simulink model "AccTarSel"  (R2018b)
settings: Solver=FixedStepDiscrete  StartTime=0.0  StopTime=inf  FixedStep=0.01  RelTol=1e-3
PostLoadFcn:
  | if any(exist('dsrtsu_mdlpostloadfcn', 'file') ~= 0), dsrtsu_mdlpostloadfcn('Execute', bdroot); end
values from neighbouring files (symbols this model uses):
  P_adtMaxBDC = 1.0    [AccTarSel.sldd]
  P_aFOCApproachIntpAcitve = -0.6    [AccTarSel.sldd]
  P_aFOCApproachIntpEnsure = -1.8    [AccTarSel.sldd]
  P_CutInEnable = 1.0    [AccTarSel.sldd]
  P_dAimMin = 4.5    [AccTarSel.sldd]
  P_dAimMinAVP = 1.5    [AccTarSel.sldd]
  P_dObjDrvOffMax = 5.0    [AccTarSel.sldd]
  P_dObjDrvOffMin = 3.0    [AccTarSel.sldd]
  P_dObjLowHystDecToStop = 4.5    [AccTarSel.sldd]
  P_dObjLowHystDecToStopAVP = 1.5    [AccTarSel.sldd]
  P_dObjUpperHystDecToStop = 5.0    [AccTarSel.sldd]
  P_dResMax = 5.0    [AccTarSel.sldd]
  P_dStandStill = 3.0    [AccTarSel.sldd]
  P_dStandStillMin = 2.0    [AccTarSel.sldd]
  P_dvarYMax4PO = 1.0    [AccTarSel.sldd]
  P_dyCutInThres = 3.6    [AccTarSel.sldd]
  P_facBDCInit = 0.7    [AccTarSel.sldd]
  P_facBDCIterCalc = 0.8    [AccTarSel.sldd]
  P_facFOCNegDiff = 0.3    [AccTarSel.sldd]
  P_facFOCPosDiff = 0.2    [AccTarSel.sldd]
  P_kapHystThres = 0.0005    [AccTarSel.sldd]
  P_PlausIntegDisable = 0.0    [AccTarSel.sldd]
  P_plausMin4PO = 0.5    [AccTarSel.sldd]
  P_probExistMin4PO = 0.8    [AccTarSel.sldd]
  P_StandObjEnable = 0.0    [AccTarSel.sldd]
  P_tAxTrackNegLower = 0.3    [AccTarSel.sldd]
  P_tAxTrackNegUpper = 0.6    [AccTarSel.sldd]
  P_tAxTrackPosLower = 1.0    [AccTarSel.sldd]
  P_tAxTrackPosUpper = 2.0    [AccTarSel.sldd]
  P_tBDCStartFilt = 0.2    [AccTarSel.sldd]
  P_tCSC = 3.5    [AccTarSel.sldd]
  P_tCurvFilt = 0.2    [AccTarSel.sldd]
  P_tCutInFilt = 0.5    [AccTarSel.sldd]
  P_tFiltAxAbsPONegFast = 0.1    [AccTarSel.sldd]
  P_tFiltAxAbsPONegSlow = 0.4    [AccTarSel.sldd]
  P_tFiltAxAbsPOPosFast = 1.2    [AccTarSel.sldd]
  P_tFiltAxAbsPOPosSlow = 2.0    [AccTarSel.sldd]
  P_tFiltAxAbsPOStand = 2.0    [AccTarSel.sldd]
  P_tFiltDAim = 0.1    [AccTarSel.sldd]
  P_tFiltDsd = 0.1    [AccTarSel.sldd]
  P_tFiltSpdLim = 3.0    [AccTarSel.sldd]
  P_tFiltVxAxPOFast = 0.15    [AccTarSel.sldd]
  P_tFiltVxAxPOSlow = 0.25    [AccTarSel.sldd]
  P_tFOCStatAccelFast = 4.0    [AccTarSel.sldd]
  P_tFOCStatAccelSlow = 3.5    [AccTarSel.sldd]
  P_tFOCStatDecelFast = 4.0    [AccTarSel.sldd]
  P_tFOCStatDecelSlow = 3.2    [AccTarSel.sldd]
  P_tMinDrvPhase = 2.0    [AccTarSel.sldd]
  P_tPredObjLeav = 1.2    [AccTarSel.sldd]
  P_tRollingFilt = 0.5    [AccTarSel.sldd]
  P_tRollingFinFilt = 1.0    [AccTarSel.sldd]
  P_tSSCNeg = 4.5    [AccTarSel.sldd]
  P_tSSCPos = 5.5    [AccTarSel.sldd]
  P_tToStop = 5.0    [AccTarSel.sldd]
  P_tToStopInBDC = 6.0    [AccTarSel.sldd]
  P_tToStopTrig = 4.0    [AccTarSel.sldd]
  P_vEgoDecToStop = 3.0    [AccTarSel.sldd]
  P_vEgoLowBDC = 4.0    [AccTarSel.sldd]
  P_vFOCNegDiff = 4.0    [AccTarSel.sldd]
  P_vFOCPosDiff = 5.0    [AccTarSel.sldd]
  P_vFOCStationaryFast = 15.0    [AccTarSel.sldd]
  P_vFOCStationarySlow = 5.0    [AccTarSel.sldd]
  P_vObjDrvOff = 0.5    [AccTarSel.sldd]
  P_vObjLowHystDecToStop = 0.5    [AccTarSel.sldd]
  P_vObjNoStop = 1.0    [AccTarSel.sldd]
  P_vObjReCalc = 1.0    [AccTarSel.sldd]
  P_vObjStop = 0.3    [AccTarSel.sldd]
  P_vObjUpperHystDecToStop = 0.8    [AccTarSel.sldd]
  P_vStandStill = 0.3    [AccTarSel.sldd]
  P_vStandStillHyst = 0.3    [AccTarSel.sldd]
  P_vyCutInThres = 0.5    [AccTarSel.sldd]
libraries: simulink x21, LPFilter x12
(part 9 of 11)

== system AccTarSel/ACC_Control/FollowObjCtrl/FollowObjValid/StationaryCtrl/If Action Subsystem2 ==
  Action Port : ActionPort  ActionType=else
  Constant : Constant  Value=0  OutDataTypeStr=single
  Out1 : Outport
  wires:
  Constant/1 -> Out1/1

== system AccTarSel/ACC_Control/FollowObjCtrl/FollowObjValid/StationaryCtrl/If Action Subsystem4 ==
  vRelAim : Inport
  vRel : Inport  Port=2
  Action Port : ActionPort  ActionType=elseif
  Add : Sum  Inputs=+-
  Out1 : Outport
  wires:
  Add/1 -> Out1/1
  vRel/1 -> Add/2
  vRelAim/1 -> Add/1

== system AccTarSel/ACC_Control/FollowObjCtrl/FollowObjValid/StationaryCtrl/calcCharactVal ==
  note: When dx>dAim, characteristic curve should be divided into 2 segment
      | to avoid constant low speed approaching in far-away case.
  <dx> : Inport
  dAim : Inport  Port=2
  Add1 : Sum  Inputs=+-
  Add2 : Sum
  Divide : Product  Inputs=*/
  Divide1 : Product  Inputs=*/
  If : If  NumInputs=3  IfExpression=u1 == 1  ElseIfExpressions=u2 == 1,u3 == 1
  If Action Subsystem : Subsystem  TreatAsAtomicUnit=on
  If Action Subsystem4 : Subsystem  TreatAsAtomicUnit=on
  If Action Subsystem5 : Subsystem  TreatAsAtomicUnit=on
  If Action Subsystem6 : Subsystem  TreatAsAtomicUnit=on
  Merge1 : Merge  Inputs=4
  Merge2 : Merge  Inputs=4
  Min : MinMax  Inputs=2
  P_facFOCNegDiff : Constant  Value=P_facFOCNegDiff
  P_facFOCPosDiff : Constant  Value=P_facFOCPosDiff
  P_vFOCNegDiff : Constant  Value=P_vFOCNegDiff
  P_vFOCPosDiff : Constant  Value=P_vFOCPosDiff
  Relational Operator : RelationalOperator  Operator=<  OutDataTypeStr=boolean  RndMeth=Simplest
  Relational Operator1 : RelationalOperator  Operator=<  OutDataTypeStr=boolean  RndMeth=Simplest
  Relational Operator2 : RelationalOperator  Operator=<  OutDataTypeStr=boolean  RndMeth=Simplest
  vUpper : Outport
  vLower : Outport  Port=2
  wires:
  dAim/1 -> If Action Subsystem5/2(dAim), If Action Subsystem4/2(dAim), Add2/1, Relational Operator1/2, Add1/1, Min/1
  P_facFOCPosDiff/1 -> Divide1/2
  <dx>/1 -> Relational Operator2/1, If Action Subsystem/1(dActual), If Action Subsystem6/1(dActual), If Action Subsystem5/1(dActual), If Action Subsystem4/1(dActual), Relational Operator1/1, Relational Operator/1
  Relational Operator1/1 -> If/2
  Min/1 -> Add1/2  "dThresNeg"
  Add2/1 -> If Action Subsystem6/2(dBPPos), Relational Operator2/2  "dBreakPointPos"
  If Action Subsystem5/1(vUpper) -> Merge1/3
  If/3 -> If Action Subsystem5/Action
  If Action Subsystem/1(vUpper) -> Merge1/1
  Divide/1 -> Min/2
  Add1/1 -> Relational Operator/2, If Action Subsystem/2(dBPNeg)  "dBreakPointNeg"
  P_facFOCNegDiff/1 -> Divide/2
  If/1 -> If Action Subsystem/Action
  Merge2/1 -> vLower/1
  Divide1/1 -> Add2/2
  Relational Operator/1 -> If/1
  If/2 -> If Action Subsystem4/Action
  Merge1/1 -> vUpper/1
  P_vFOCPosDiff/1 -> Divide1/1
  If Action Subsystem5/2(vLower) -> Merge2/3
  If Action Subsystem6/1(vUpper) -> Merge1/4
  If Action Subsystem6/2(vLower) -> Merge2/4
  P_vFOCNegDiff/1 -> Divide/1
  If Action Subsystem4/2(vLower) -> Merge2/2
  Relational Operator2/1 -> If/3
  If/4 -> If Action Subsystem6/Action
  If Action Subsystem4/1(vUpper) -> Merge1/2
  If Action Subsystem/2(vLower) -> Merge2/1

== system AccTarSel/ACC_Control/FollowObjCtrl/FollowObjValid/StopGoCtrl/If Action Subsystem ==
  In1 : Inport
  Action Port : ActionPort  ActionType=then
  Out1 : Outport
  wires:
  In1/1 -> Out1/1

== system AccTarSel/ACC_Control/FollowObjCtrl/FollowObjValid/StopGoCtrl/If Action Subsystem1 ==
  In1 : Inport
  Action Port : ActionPort  ActionType=elseif
  Out1 : Outport
  wires:
  In1/1 -> Out1/1

== system AccTarSel/ACC_Control/FollowObjCtrl/FollowObjValid/StopGoCtrl/If Action Subsystem2 ==
  In1 : Inport
  Action Port : ActionPort  ActionType=else
  Out1 : Outport
  wires:
  In1/1 -> Out1/1

== system AccTarSel/ACC_Target_Selection/Subsystem/ValidObjCalc/CutInCalc/If Action Subsystem ==
  Action Port : ActionPort  ActionType=else
  Constant : Constant  Value=0  OutDataTypeStr=single
  Out1 : Outport
  Out2 : Outport  Port=2
  Out3 : Outport  Port=3
  wires:
  Constant/1 -> Out3/1, Out2/1, Out1/1

== system AccTarSel/ACC_Target_Selection/Subsystem/ValidObjCalc/CutInCalc/Subsystem ==
  objInfo : Inport
  ATS_Internal_K1 : Inport  Port=2
  dyToTraj : Inport  Port=3
  SYS_Info_st : Inport  Port=4
  Action Port : ActionPort  ActionType=then
  Bus Selector : BusSelector  OutputSignals=ID,vy,MotionSts
  Bus Selector1 : BusSelector  OutputSignals=ID,probCutInFilt
  If : If  IfExpression=u1 == 1
  If Action Subsystem : Subsystem  TreatAsAtomicUnit=on
  Merge : Merge
  Merge1 : Merge
  Merge2 : Merge
  Relational Operator3 : RelationalOperator  Operator===  OutDataTypeStr=boolean  RndMeth=Simplest
  Subsystem : Subsystem
  probCutInFilt : Outport
  dyCutInPred : Outport  Port=2
  probCutInRaw : Outport  Port=3
  wires:
  objInfo/1 -> Bus Selector/1
  ATS_Internal_K1/1 -> Bus Selector1/1
  Bus Selector1/1 -> Relational Operator3/1  "<ID>"
  Bus Selector/1 -> Relational Operator3/2  "<ID>"
  dyToTraj/1 -> If Action Subsystem/1(In1), Subsystem/2(dyToTraj)
  Bus Selector/2 -> Subsystem/3(<vy>)  "<vy>"
  Relational Operator3/1 -> If/1
  If/1 -> Subsystem/Action
  If/2 -> If Action Subsystem/Action
  Bus Selector1/2 -> Subsystem/1(probCutInK1)  "<probCutInFilt>"
  Subsystem/1(probCutInFilt) -> Merge/1
  If Action Subsystem/1(probCutInFiltInit) -> Merge/2
  If Action Subsystem/2(dyCutInPredInit) -> Merge1/2
  Subsystem/2(dyCutInPred) -> Merge1/1
  Merge1/1 -> dyCutInPred/1  "dyCutInPred"
  Merge/1 -> probCutInFilt/1  "probCutInFilt"
  SYS_Info_st/1 -> Subsystem/5(SYS_Info_st)
  Subsystem/3(probCutInRaw) -> Merge2/1
  If Action Subsystem/3(probCutInRawInit) -> Merge2/2
  Merge2/1 -> probCutInRaw/1  "probCutInRaw"
  Bus Selector/3 -> Subsystem/4(MotionSts)  "<MotionSts>"

== system AccTarSel/ACC_Target_Selection/Subsystem/ValidObjCalc/EgoCourseDeviation/DistanceToTraj ==
  In1 : Inport
  In2 : Inport  Port=2
  In3 : Inport  Port=3
  Action Port : ActionPort  ActionType=then
  Add : Sum  Inputs=++++
  Add1 : Sum  Inputs=+-
  Bus Selector : BusSelector  OutputSignals=a,b,c,d
  Constant : Constant  Value=3  OutDataTypeStr=single
  Multiply : Product
  Multiply1 : Product
  Multiply2 : Product
  Square : Math  Operator=pow  SaturateOnIntegerOverflow=on
  Square1 : Math  Operator=square  SaturateOnIntegerOverflow=on
  Out1 : Outport
  wires:
  In1/1 -> Multiply2/1, Square1/1, Square/1
  Constant/1 -> Square/2
  Square/1 -> Multiply/1
  Bus Selector/1 -> Multiply/2  "<a>"
  Square1/1 -> Multiply1/1
  Bus Selector/2 -> Multiply1/2  "<b>"
  Bus Selector/3 -> Multiply2/2  "<c>"
  Multiply/1 -> Add/1
  Multiply1/1 -> Add/2
  In3/1 -> Bus Selector/1
  In2/1 -> Add1/1
  Add1/1 -> Out1/1
  Multiply2/1 -> Add/3
  Bus Selector/4 -> Add/4  "<d>"
  Add/1 -> Add1/2

== system AccTarSel/ACC_Target_Selection/Subsystem/ValidObjCalc/EgoCourseDeviation/If Action Subsystem ==
  In1 : Inport
  Action Port : ActionPort  ActionType=else
  Out1 : Outport
  wires:
  In1/1 -> Out1/1

== system AccTarSel/ACC_Target_Selection/Subsystem/ValidObjCalc/LanePlausCalc/If Action Subsystem ==
  In1 : Inport
  Action Port : ActionPort  ActionType=then
  Out1 : Outport
  wires:
  In1/1 -> Out1/1

== system AccTarSel/ACC_Target_Selection/Subsystem/ValidObjCalc/LanePlausCalc/If Action Subsystem1 ==
  In1 : Inport
  Action Port : ActionPort  ActionType=else
  Out1 : Outport
  wires:
  In1/1 -> Out1/1

== system AccTarSel/ACC_Target_Selection/Subsystem/ValidObjCalc/LaneProbCalc/If Action Subsystem ==
  In1 : Inport
  Action Port : ActionPort  ActionType=else
  Out1 : Outport
  wires:
  In1/1 -> Out1/1

== system AccTarSel/ACC_Target_Selection/Subsystem/ValidObjCalc/LaneProbCalc/Subsystem ==
  <dx> : Inport
  ID : Inport  Port=2
  In2 : Inport  Port=3
  ATS_Internal_K1 : Inport  Port=4
  Action Port : ActionPort  ActionType=then
  1-D Lookup Table : Lookup_n-D  NumberOfTableDimensions=1  LookupTableObject=''  BreakpointsForDimension1=[0,20,40]  BreakpointsForDimension1FirstPoint=10  BreakpointsForDimension2FirstPoint=10  BreakpointsForDimension1Spacing=12  BreakpointsForDimension2Spacing=12  IndexSearchMethod=Linear search  Table=[1.6,1.6,1.8]  ExtrapMethod=Clip  InternalRulePriority=Speed  RndMeth=Simplest  InputSameDT=on
  1-D Lookup Table1 : Lookup_n-D  NumberOfTableDimensions=1  LookupTableObject=''  BreakpointsForDimension1=[-0.2,0.2]  BreakpointsForDimension1FirstPoint=10  BreakpointsForDimension2FirstPoint=10  BreakpointsForDimension1Spacing=12  BreakpointsForDimension2Spacing=12  IndexSearchMethod=Linear search  Table=[-1,1.2]  ExtrapMethod=Clip  InternalRulePriority=Speed  RndMeth=Simplest  InputSameDT=on
  AND : Logic  AllPortsSameDT=off  OutDataTypeStr=boolean
  Abs : Abs
  Add : Sum  Inputs=+-
  Add1 : Sum
  Bus Selector : BusSelector  OutputSignals=ID,ValidEgoLane
  Constant : Constant  Value=0.15  OutDataTypeStr=single
  Constant1 : Constant  Value=0  OutDataTypeStr=single
  Divide : Product  Inputs=*/
  Relational Operator : RelationalOperator  Operator===  OutDataTypeStr=boolean  RndMeth=Simplest
  Switch : Switch  Criteria=u2 > Threshold
  probEgoTraj : Outport
  wires:
  <dx>/1 -> 1-D Lookup Table/1
  Add1/1 -> Divide/2, Add/1  "dyWidthTraj"
  Add/1 -> Divide/1
  Divide/1 -> 1-D Lookup Table1/1
  1-D Lookup Table1/1 -> probEgoTraj/1  "probEgoTraj"
  Abs/1 -> Add/2  "dyToTrajAbs"
  In2/1 -> Abs/1
  ATS_Internal_K1/1 -> Bus Selector/1
  Bus Selector/1 -> Relational Operator/2  "<ID>"
  ID/1 -> Relational Operator/1
  Relational Operator/1 -> AND/1
  Bus Selector/2 -> AND/2  "<ValidEgoLane>"
  AND/1 -> Switch/2
  Constant/1 -> Switch/1
  Constant1/1 -> Switch/3
  1-D Lookup Table/1 -> Add1/2
  Switch/1 -> Add1/1

== system AccTarSel/ACC_Target_Selection/Subsystem/ValidObjCalc/TargetPlausCheck/If Action Subsystem ==
  In1 : Inport
  Action Port : ActionPort  ActionType=else
  Out1 : Outport
  wires:
  In1/1 -> Out1/1

== system AccTarSel/ACC_Target_Selection/Subsystem/ValidObjCalc/TargetPlausCheck/Subsystem ==
  fus_objdata_st : Inport
  VSI_VehState_st : Inport  Port=2
  plausibility : Inport  Port=3
  Action Port : ActionPort  ActionType=then
  CheckExistence : Subsystem
  CheckFOV : Subsystem
  CheckMotSts : Subsystem
  CheckPlaus : Subsystem
  Logical Operator : Logic  Inputs=4  AllPortsSameDT=off  OutDataTypeStr=boolean
  Out1 : Outport
  wires:
  VSI_VehState_st/1 -> CheckFOV/2(In2)
  CheckMotSts/1(Out1) -> Logical Operator/2
  fus_objdata_st/1 -> CheckExistence/1(In1), CheckMotSts/1(In1), CheckFOV/1(In1)
  plausibility/1 -> CheckPlaus/1(In1)
  CheckPlaus/1(Out1) -> Logical Operator/4
  CheckFOV/1(Out1) -> Logical Operator/1
  CheckExistence/1(Out1) -> Logical Operator/3
  Logical Operator/1 -> Out1/1

== system AccTarSel/RTI Data/RTI Data Store/RTI Data Store/RTI Data Store/RTI Data Store ==

== system AccTarSel/ACC_Control/FollowObjCtrl/FollowObjValid/ApproachingCtrl/case1/Subsystem ==
  vObjRel : Inport
  dSlowDown : Inport  Port=2
  aAbsObj : Inport  Port=3
  Action Port : ActionPort  ActionType=else
  Abs : Abs
  Add : Sum
  Add1 : Sum  Inputs=+-
  Constant : Constant  Value=2  OutDataTypeStr=single
  Constant1 : Constant  Value=0  OutDataTypeStr=single
  Constant2 : Constant  Value=255  OutDataTypeStr=single
  Divide : Product  Inputs=*/
  Divide1 : Product  Inputs=*/
  Min : MinMax  Inputs=2
  Multiply : Product
  Square1 : Math  Operator=square  SaturateOnIntegerOverflow=on
  tSameSpd : Outport
  aRel : Outport  Port=2
  wires:
  Divide1/1 -> Abs/1
  Constant1/1 -> Add1/1
  Square1/1 -> Add1/2
  Add1/1 -> Divide/1
  Constant/1 -> Multiply/2
  Multiply/1 -> Divide/2
  Divide/1 -> Add/1, Divide1/2
  Add/1 -> aRel/1
  dSlowDown/1 -> Multiply/1
  vObjRel/1 -> Square1/1, Divide1/1
  aAbsObj/1 -> Add/2
  Abs/1 -> Min/2
  Constant2/1 -> Min/1
  Min/1 -> tSameSpd/1

== system AccTarSel/ACC_Control/FollowObjCtrl/FollowObjValid/ApproachingCtrl/case1/Subsystem1 ==
  aAbsObj : Inport
  Action Port : ActionPort  ActionType=then
  Constant : Constant  Value=255  OutDataTypeStr=single
  tSameSpd : Outport
  aRel : Outport  Port=2
  wires:
  Constant/1 -> tSameSpd/1
  aAbsObj/1 -> aRel/1

== system AccTarSel/ACC_Control/FollowObjCtrl/FollowObjValid/ApproachingCtrl/isObjLeaving/Approaching ==
  Action Port : ActionPort  ActionType=then
  Constant : Constant  Value=0  OutDataTypeStr=boolean
  Out1 : Outport
  wires:
  Constant/1 -> Out1/1

== system AccTarSel/ACC_Control/FollowObjCtrl/FollowObjValid/ApproachingCtrl/isObjLeaving/Hold ==
  In1 : Inport
  Action Port : ActionPort  ActionType=else
  Out1 : Outport
  wires:
  In1/1 -> Out1/1

== system AccTarSel/ACC_Control/FollowObjCtrl/FollowObjValid/ApproachingCtrl/isObjLeaving/Leaving ==
  Action Port : ActionPort  ActionType=elseif
  Constant : Constant  OutDataTypeStr=boolean
  Out1 : Outport
  wires:
  Constant/1 -> Out1/1

== system AccTarSel/ACC_Control/FollowObjCtrl/FollowObjValid/BrakeDistCtrl/calcA/If Action Subsystem ==
  Profile : Inport
  tElapse : Inport  Port=2
  dRes : Inport  Port=3
  SYS_Info_st : Inport  Port=4
  Action Port : ActionPort  ActionType=then
  Bus Selector : BusSelector  OutputSignals=T30,T,a0,adt1,aMax,adt2,SmoothStopCond,a0Raw
  If : If  NumInputs=2  IfExpression=u1 == 1  ElseIfExpressions=u2 == 1
  If Action Subsystem : Subsystem  TreatAsAtomicUnit=on
  If Action Subsystem1 : Subsystem  TreatAsAtomicUnit=on
  If Action Subsystem2 : Subsystem  TreatAsAtomicUnit=on
  If Action Subsystem3 : Subsystem  TreatAsAtomicUnit=on
  If1 : If  IfExpression=u1 == 1
  Memory : Memory
  Memory1 : Memory  InheritSampleTime=on
  Merge : Merge  Inputs=3
  Merge1 : Merge
  Relational Operator : RelationalOperator  Operator=<=  OutDataTypeStr=boolean  RndMeth=Simplest
  Relational Operator1 : RelationalOperator  Operator=<=  OutDataTypeStr=boolean  RndMeth=Simplest
  Subsystem : Subsystem
  Out1 : Outport
  wires:
  Profile/1 -> Bus Selector/1
  tElapse/1 -> [tElapse], If Action Subsystem1/1(t), If Action Subsystem/1(t), Relational Operator1/1, Relational Operator/1
  Bus Selector/1 -> If Action Subsystem1/4(T30), Relational Operator/2  "<T30>"
  Relational Operator/1 -> If/1
  Bus Selector/3 -> If Action Subsystem/2(a0)  "<a0>"
  Bus Selector/4 -> If Action Subsystem/3(adt1)  "<adt1>"
  Bus Selector/2 -> Relational Operator1/2  "<T>"
  Relational Operator1/1 -> If/2
  If/1 -> If Action Subsystem/Action
  If/2 -> If Action Subsystem1/Action
  Bus Selector/5 -> If Action Subsystem1/2(aMax)  "<aMax>"
  Bus Selector/6 -> If Action Subsystem1/3(adt2)  "<adt2>"
  If/3 -> If Action Subsystem2/Action
  If Action Subsystem/1(Out1) -> Merge/1
  If Action Subsystem1/1(Out1) -> Merge/2
  If Action Subsystem2/1(Out1) -> Merge/3
  Bus Selector/7 -> [SmoothStopCond]  "<SmoothStopCond>"
  [SmoothStopCond] -> If1/1
  Bus Selector/8 -> [a0Raw]  "<a0Raw>"
  Merge/1 -> Memory/1, If Action Subsystem3/1(In1), Subsystem/1(aCharact)  "aCharact"
  [a0Raw] -> Subsystem/2(a0Raw)
  [tElapse] -> Subsystem/3(tElapse)
  If1/1 -> If Action Subsystem3/Action
  If1/2 -> Subsystem/Action
  If Action Subsystem3/1(Out1) -> Merge1/1
  Subsystem/1(Out1) -> Merge1/2
  Merge1/1 -> Memory1/1, Out1/1  "aBDC"
  dRes/1 -> If Action Subsystem1/5(dRes)
  Memory/1 -> If Action Subsystem1/6(aCharactK1)
  SYS_Info_st/1 -> Subsystem/4(SYS_Info_st), If Action Subsystem1/7(SYS_Info_st)
  Memory1/1 -> Subsystem/5(aBDCK1)

== system AccTarSel/ACC_Control/FollowObjCtrl/FollowObjValid/BrakeDistCtrl/calcA/If Action Subsystem1 ==
  Action Port : ActionPort  ActionType=else
  Constant : Constant  Value=0  OutDataTypeStr=single
  Out1 : Outport
  wires:
  Constant/1 -> Out1/1

== system AccTarSel/ACC_Control/FollowObjCtrl/FollowObjValid/BrakeDistCtrl/calcCriteria/calcObjStop ==
  vAbsObj : Inport
  aAbsObj : Inport  Port=2
  BDC_StateK1 : Inport  Port=3
  AND : Logic  AllPortsSameDT=off  OutDataTypeStr=boolean
  Bus Creator : BusCreator  Inputs=3
  Constant6 : Constant  Value=0.5  OutDataTypeStr=single
  If : If  NumInputs=2  IfExpression=u1 == 1  ElseIfExpressions=u2 == 1
  Merge : Merge  Inputs=3
  Merge1 : Merge  Inputs=3
  ObjNoStop : Subsystem  TreatAsAtomicUnit=on
  ObjStopped : Subsystem  TreatAsAtomicUnit=on
  ObjStopping : Subsystem  TreatAsAtomicUnit=on
  P_tToStop : Constant  Value=P_tToStopTrig  OutDataTypeStr=single
  P_vObjNoStop : Constant  Value=P_vObjNoStop  OutDataTypeStr=single
  P_vObjStop : Constant  Value=P_vObjStop  OutDataTypeStr=single
  Relational Operator1 : RelationalOperator  Operator=<  OutDataTypeStr=boolean  RndMeth=Simplest
  Relational Operator2 : RelationalOperator  Operator=<  OutDataTypeStr=boolean  RndMeth=Simplest
  Relational Operator3 : RelationalOperator  Operator=<  OutDataTypeStr=boolean  RndMeth=Simplest
  Relational Operator4 : RelationalOperator  Operator=>  OutDataTypeStr=boolean  RndMeth=Simplest
  Relational Operator5 : RelationalOperator  Operator=>  OutDataTypeStr=boolean  RndMeth=Simplest
  Subsystem : Subsystem
  To Workspace : ToWorkspace  VariableName=simout3  SaveFormat=Timeseries  SampleTime=-1
  ObjToStop : Outport
  ObjToStopTrig : Outport  Port=2
  dObjToStop : Outport  Port=3
  wires:
  vAbsObj/1 -> Bus Creator/1, Relational Operator4/1, ObjStopping/1(vAbsObj), Relational Operator2/1
  Merge/1 -> Bus Creator/3, Relational Operator3/1, Relational Operator1/1  "tToStop"
  P_tToStop/1 -> Relational Operator3/2
  aAbsObj/1 -> Bus Creator/2, Relational Operator5/1, ObjStopping/2(aAbsObj)
  Merge1/1 -> dObjToStop/1  "dObjToStop"
  Subsystem/1(tStop) -> Relational Operator1/2
  Relational Operator1/1 -> ObjToStop/1
  Relational Operator3/1 -> ObjToStopTrig/1
  P_vObjStop/1 -> Relational Operator2/2
  ObjStopped/1(tToStop) -> Merge/1
  ObjStopping/1(tToStop) -> Merge/2
  ObjNoStop/1(tToStop) -> Merge/3
  ObjStopped/2(dToStop) -> Merge1/1
  ObjStopping/2(dToStop) -> Merge1/2
  ObjNoStop/2(dToStop) -> Merge1/3
  P_vObjNoStop/1 -> Relational Operator4/2
  Constant6/1 -> Relational Operator5/2
  Relational Operator4/1 -> AND/1
  Relational Operator5/1 -> AND/2
  AND/1 -> If/1
  If/1 -> ObjNoStop/Action
  Relational Operator2/1 -> If/2
  If/2 -> ObjStopped/Action
  If/3 -> ObjStopping/Action
  Bus Creator/1 -> To Workspace/1
  BDC_StateK1/1 -> Subsystem/1(StateK1)
